simulink library "schmehlTangentRotation_ul"  (R2018b)
settings: Solver=VariableStepAuto  StartTime=0.0  StopTime=10.0  RelTol=1e-3
libraries: sharedutil x1
settings Model: Creator=jldanie5  LastModifiedBy=jldanie5

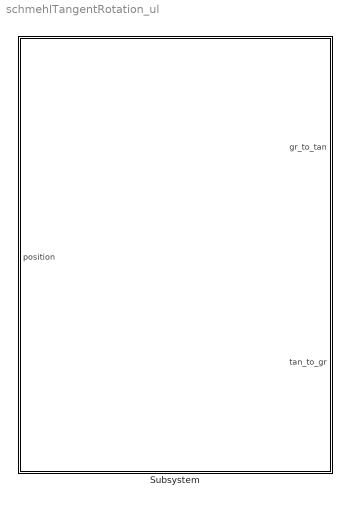
== system schmehlTangentRotation_ul ==
  Subsystem : Subsystem

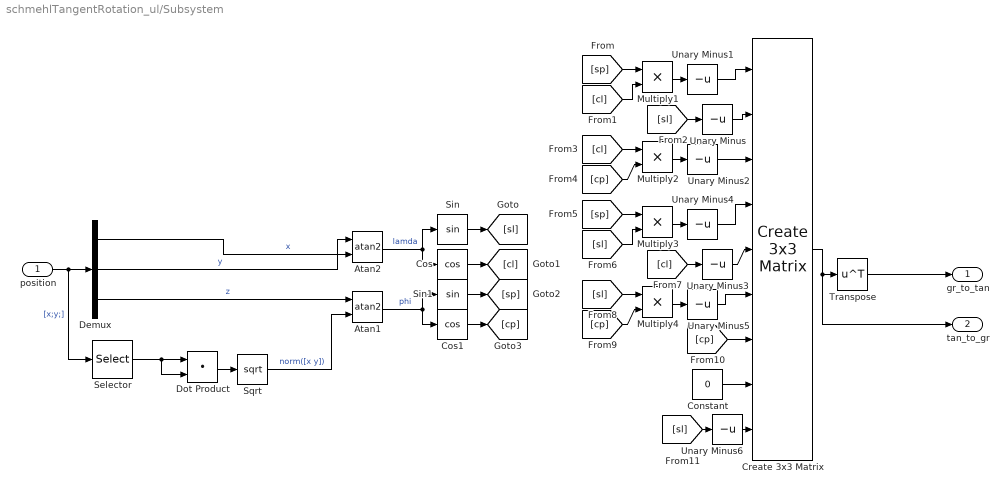
== system schmehlTangentRotation_ul/Subsystem ==
  position : Inport
  Atan1 : Trigonometry  Operator=atan2
  Atan2 : Trigonometry  Operator=atan2
  Constant : Constant  Value=0
  Cos : Trigonometry  Operator=cos
  Cos1 : Trigonometry  Operator=cos
  Create 3x3 Matrix : sharedutil/Create 3x3 Matrix  aMode=aMode
  Demux : Demux  Outputs=3
  Dot Product : DotProduct  InputSameDT=on  OutDataTypeStr=Inherit: Inherit via internal rule
  Multiply{1..4} (4 alike) : Product
  Selector : Selector  InputPortWidth=3  IndexOptions=Index vector (dialog)  Indices=[1 2]  OutputSizes=1
  Sin : Trigonometry
  Sin1 : Trigonometry
  Sqrt : Sqrt  SaturateOnIntegerOverflow=on
  Transpose : Math  Operator=transpose  SaturateOnIntegerOverflow=on
  Unary Minus{,1..6} (7 alike) : UnaryMinus
  gr_to_tan : Outport
  tan_to_gr : Outport  Port=2
  wires:
  position/1 -> Selector/1, Demux/1  "[x;y;]"
  Demux/2 -> Atan2/1  "y"
  Demux/1 -> Atan2/2  "x"
  Selector/1 -> Dot Product/2, Dot Product/1
  Dot Product/1 -> Sqrt/1
  Demux/3 -> Atan1/1  "z"
  Sqrt/1 -> Atan1/2  "norm([x y])"
  Transpose/1 -> gr_to_tan/1
  Create 3x3 Matrix/1 -> tan_to_gr/1, Transpose/1
  Atan2/1 -> Cos/1, Sin/1  "lamda"
  Atan1/1 -> Cos1/1, Sin1/1  "phi"
  Sin/1 -> [sl]
  Cos/1 -> [cl]
  Sin1/1 -> [sp]
  Cos1/1 -> [cp]
  Unary Minus1/1 -> Create 3x3 Matrix/1
  [sl] -> Unary Minus/1
  Unary Minus/1 -> Create 3x3 Matrix/2
  Multiply1/1 -> Unary Minus1/1
  [sp] -> Multiply1/1
  [cl] -> Multiply1/2
  [cl] -> Multiply2/1
  [cp] -> Multiply2/2
  Multiply2/1 -> Unary Minus2/1
  Unary Minus2/1 -> Create 3x3 Matrix/3
  Unary Minus5/1 -> Create 3x3 Matrix/6
  Multiply3/1 -> Unary Minus4/1
  Unary Minus4/1 -> Create 3x3 Matrix/4
  [sp] -> Multiply3/1
  [cp] -> Multiply4/2
  Multiply4/1 -> Unary Minus5/1
  Unary Minus3/1 -> Create 3x3 Matrix/5
  [sl] -> Multiply4/1
  [cl] -> Unary Minus3/1
  [sl] -> Multiply3/2
  [cp] -> Create 3x3 Matrix/7
  Constant/1 -> Create 3x3 Matrix/8
  Unary Minus6/1 -> Create 3x3 Matrix/9
  [sl] -> Unary Minus6/1
